simulink model "EN_EVPowerFlow_AveModel"  (R2021a)
settings: Solver=ode23t  StartTime=0.0  StopTime=20  MaxStep=1e-3  RelTol=1e-3  AbsTol=1e-3
libraries: nesl_utility x15, fl_lib x13, ee_lib x9, eeGeneralControl x4, pid_lib x1
settings Model: SimulationMode=accelerator  PacingRate=1000  Creator=ykamatan  LastModifiedBy=ykamatan
settings SolverCC: AutoScaleAbsTol=off  SolverJacobianMethodControl=SparsePerturbation  DaesscMode=Fast
settings DebuggingCC: SymbolicDimsDataTypeCodeGenerationDiagnostic=none  SFMachineParentedDataDiag=warning
settings SFSimCC: CustomCodeUndefinedFunction=UseInterfaceOnly
settings SimscapeCC: SimscapeLogType=all  SimscapeLogSimulationStatistics=on  SimscapeLogDataHistory=10000

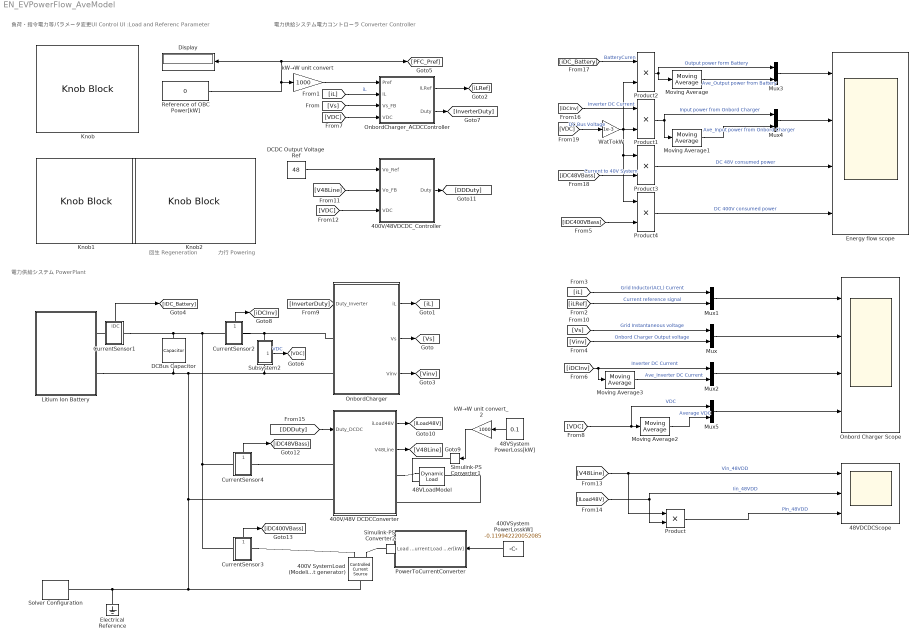
== system EN_EVPowerFlow_AveModel ==
  note: 回生
      | Regeneration
  note: 力行
      | Powering
  note: 負荷・指令電力等パラメータ変更UI
      | Control UI :Load and Referenc Parameter
  note: 電力供給システム PowerPlant
  note: 電力供給システム電力コントローラ
      | Converter Controller
  400V SystemLoad (Modeling as current generator) : fl_lib/Electrical/Electrical Sources/Controlled Current Source
  400V/48V DCDCConverter : Subsystem
  400V/48VDCDC_Controller : Subsystem
  400VSystem PowerLosskW] : Constant  Value=-0.119942220052085
  48VDCDCScope : Scope  NumInputPorts=3
  48VLoadModel : ee_lib/Passive/Dynamic Load  load_type=ee.enum.dc_ac.dc  enable_fault=ee.enum.faults.faultEnable.no  min_supply_voltage=38 V  pow_min=1e-3 W  G_reverse=1e-6 S  deltaV=1e-3 V  f0=60 Hz  Vrms_min=200 V  Pmin=1e-3 W  fault_action=ee.enum.faults.faultAction.none  t_fault=1 s  open_conductance=1e-4 S
      settings: SourceProductBaseCode=PS  InternalSimscapePortConfiguration="{\"Bottom\":[],\"Left\":[{\"id\":\"p\",\"label\":\"+\",\"type\":\"foundation.electrical.electrical\"}],\"Right\":[{\"id\":\"n\",\"label\":\"-\",\"type\":\"foundation.electrical.electrical\"}],\"Top\":[{\"id\":\"P\",\"label\":\"P\",\"type\":\"input\"}]}"
  48VSystem PowerLoss[kW] : Constant  Value=0.1
  CurrentSensor1 : Subsystem
      settings: PortSchema="{\"entries\":[{\"content\":{\"sides\":[{\"content\":{\"connectorIds\":[\"LConn1\"]},\"type\":\"ConnectorPlacement.EquallySpacedRectSide\",\"uuid\":\"7286f59e-cee0-499d-832c-cf6f33a1b017\"},{\"content\":{\"connectorIds\":[\"RConn1\"],\"side\":\"RIGHT\"},\"type\":\"ConnectorPlacement.EquallySpacedRectSide\",\"uuid\":\"6a983281-a6bc-4a57-a5ba-c4da9a8828f4\"},{\"content\":{\"connectorIds\":[\"Out1\"],\"side\":\"TOP\"},\"type\":\"ConnectorPlacement.EquallySpacedRectSide\",\"uuid\":\"6969f7e7-2dce-4d64-b6f6-e92ef9035b1a\"}]},\"type\":\"ConnectorPlacement.EquallySpacedConnector\",\"uuid\":\"05fc616a-5402-4b75-b59e-8cf259d71f3d\"}],\"packageUris\":[\"http://schema.mathworks.com/mf0/Connector/R2020b\"],\"version\":\"1.0\"}"
  CurrentSensor2 : Subsystem
      settings: PortSchema="{\"entries\":[{\"content\":{\"sides\":[{\"content\":{\"connectorIds\":[\"LConn1\"]},\"type\":\"ConnectorPlacement.EquallySpacedRectSide\",\"uuid\":\"7286f59e-cee0-499d-832c-cf6f33a1b017\"},{\"content\":{\"connectorIds\":[\"RConn1\"],\"side\":\"RIGHT\"},\"type\":\"ConnectorPlacement.EquallySpacedRectSide\",\"uuid\":\"6a983281-a6bc-4a57-a5ba-c4da9a8828f4\"},{\"content\":{\"connectorIds\":[\"Out1\"],\"side\":\"TOP\"},\"type\":\"ConnectorPlacement.EquallySpacedRectSide\",\"uuid\":\"6969f7e7-2dce-4d64-b6f6-e92ef9035b1a\"}]},\"type\":\"ConnectorPlacement.EquallySpacedConnector\",\"uuid\":\"05fc616a-5402-4b75-b59e-8cf259d71f3d\"}],\"packageUris\":[\"http://schema.mathworks.com/mf0/Connector/R2020b\"],\"version\":\"1.0\"}"
  CurrentSensor3 : Subsystem
      settings: PortSchema="{\"entries\":[{\"content\":{\"sides\":[{\"content\":{\"connectorIds\":[\"LConn1\"]},\"type\":\"ConnectorPlacement.EquallySpacedRectSide\",\"uuid\":\"7286f59e-cee0-499d-832c-cf6f33a1b017\"},{\"content\":{\"connectorIds\":[\"RConn1\"],\"side\":\"RIGHT\"},\"type\":\"ConnectorPlacement.EquallySpacedRectSide\",\"uuid\":\"6a983281-a6bc-4a57-a5ba-c4da9a8828f4\"},{\"content\":{\"connectorIds\":[\"Out1\"],\"side\":\"TOP\"},\"type\":\"ConnectorPlacement.EquallySpacedRectSide\",\"uuid\":\"6969f7e7-2dce-4d64-b6f6-e92ef9035b1a\"}]},\"type\":\"ConnectorPlacement.EquallySpacedConnector\",\"uuid\":\"05fc616a-5402-4b75-b59e-8cf259d71f3d\"}],\"packageUris\":[\"http://schema.mathworks.com/mf0/Connector/R2020b\"],\"version\":\"1.0\"}"
  CurrentSensor4 : Subsystem
      settings: PortSchema="{\"entries\":[{\"content\":{\"sides\":[{\"content\":{\"connectorIds\":[\"LConn1\"]},\"type\":\"ConnectorPlacement.EquallySpacedRectSide\",\"uuid\":\"7286f59e-cee0-499d-832c-cf6f33a1b017\"},{\"content\":{\"connectorIds\":[\"RConn1\"],\"side\":\"RIGHT\"},\"type\":\"ConnectorPlacement.EquallySpacedRectSide\",\"uuid\":\"6a983281-a6bc-4a57-a5ba-c4da9a8828f4\"},{\"content\":{\"connectorIds\":[\"Out1\"],\"side\":\"TOP\"},\"type\":\"ConnectorPlacement.EquallySpacedRectSide\",\"uuid\":\"6969f7e7-2dce-4d64-b6f6-e92ef9035b1a\"}]},\"type\":\"ConnectorPlacement.EquallySpacedConnector\",\"uuid\":\"05fc616a-5402-4b75-b59e-8cf259d71f3d\"}],\"packageUris\":[\"http://schema.mathworks.com/mf0/Connector/R2020b\"],\"version\":\"1.0\"}"
  DCBus Capacitor : ee_lib/Passive/Capacitor  cap_option=0  c=1000e-6 F  Cvec=[1e-05, 1e-06] F  Vvec=[0, 10] V  CV_table_symmetry=1  f_vec=[1, 10] kHz  DFext_vec=[.8, 1.2]  C_tol=5  enable_C_tol=0  tol_distribution=1  nSigma=4  r=1e-6 Ohm  g=0 1/Ohm  averaging_period=0 s  enable_operating_limits=0  operating_limit_action=2  max_working_voltage_range=[-25, 25] V  power_rating=1 W  enable_faults=0  fault_action=1  Cscale_faulted=100  R_faulted=1e-3 Ohm  G_faulted=0 1/Ohm  tau_fault=1e-3 s  enable_temporal_fault=0  t_fault=1 s  enable_behavioral_fault=0  max_permissible_voltage_range=[-100, 100] V  t_fail_on_voltage=1 s  i_specify=off  i_priority=None  i=0 A  i_nominal_specify=off  i_nominal_unit=A  i_nominal_value=1  v_specify=off  v_priority=None  v=400 V  v_nominal_specify=off  v_nominal_unit=V  v_nominal_value=1  vc_specify=on  vc_priority=High  vc=400 V  vc_nominal_specify=off  vc_nominal_unit=V  vc_nominal_value=1
  DCDC Output Voltage Ref : Constant  Value=48
  Display : Display
  Electrical Reference : fl_lib/Electrical/Electrical Elements/Electrical Reference
  Energy flow scope : Scope  NumInputPorts=4
  Knob : KnobBlock  ScaleMax=3
  Knob1 : KnobBlock  ScaleMin=0.1  ScaleMax=2
  Knob2 : KnobBlock  ScaleMin=-20  ScaleMax=20  TickInterval=2
  Litium Ion Battery : Subsystem
  Moving Average : eeGeneralControl/Moving Average  VariantControl=Variant1  LabelModeActiveChoice=Discrete  f=120  x0=0  Ts=1/120/10
      settings: SourceProductBaseCode=PS
  Moving Average1 : eeGeneralControl/Moving Average  VariantControl=Variant1  LabelModeActiveChoice=Discrete  f=120  x0=0  Ts=1/120/10
      settings: SourceProductBaseCode=PS
  Moving Average2 : eeGeneralControl/Moving Average  VariantControl=Variant1  LabelModeActiveChoice=Discrete  f=120  x0=400  Ts=1/120/10
      settings: SourceProductBaseCode=PS
  Moving Average3 : eeGeneralControl/Moving Average  VariantControl=Variant1  LabelModeActiveChoice=Discrete  f=120  x0=0  Ts=1/120/10
      settings: SourceProductBaseCode=PS
  Mux{,1..5} (6 alike) : Mux  Inputs=2
  Onbord Charger Scope : Scope  NumInputPorts=4
  OnbordCharger : Subsystem
  OnbordCharger_ACDCController : Subsystem
  PowerToCurrentConverter : Subsystem
  Product{,1..4} (5 alike) : Product
  Reference of OBC Power[kW] : Constant  Value=0
  Simulink-PS Converter1 : nesl_utility/Simulink-PS Converter  PhysicalDomain=network_engine_domain  SubClassName=ps_input  LeftPortType=input  RightPortType=output  PseudoPeriodic=off  Frequencies=[]  NoiseDistribution=none  NoiseParameters=[]  Unit=1  AffineConversion=off  FilteringAndDerivatives=provide  SimscapeFilterOrder=1  InputFilterTimeConstant=0.001  UdotUserProvided=0
      settings: SourceProductBaseCode=PW,SS
  Simulink-PS Converter2 : nesl_utility/Simulink-PS Converter  PhysicalDomain=network_engine_domain  SubClassName=ps_input  LeftPortType=input  RightPortType=output  PseudoPeriodic=off  Frequencies=[]  NoiseDistribution=none  NoiseParameters=[]  Unit=1  AffineConversion=off  FilteringAndDerivatives=provide  SimscapeFilterOrder=1  InputFilterTimeConstant=0.001  UdotUserProvided=0
      settings: SourceProductBaseCode=PW,SS
  Solver Configuration : nesl_utility/Solver Configuration  PhysicalDomain=network_engine_domain  SubClassName=solver  LeftPortType=input  RightPortType=generic  Tones=[]  Harmonics=[]  SimulateNoise=off  Profile=off  UseLocalSampling=off  EnableSwitchedLinearOptims=on  FrequencyDomain=off  UseCCode=off  RelTol=0.001  AbsTol=1e-06  MinStep=1e-09  ToWorkspace=off  RevertToSquareIcSolve=off  NumHomotopyIterations=100  PhasorMode=off  PhasorModeNumHarmonics=1  DoDC=off  ResidualTolerance=1e-09  UseLocalSolver=off  LocalSolverChoice=NE_BACKWARD_EULER_ADVANCER  LocalSolverSampleTime=0.001  DoFixedCost=off  MaxNonlinIter=3  MaxModeIter=2  ComputeImpulses=off  ImpulseIterations=2  LinearAlgebra=auto  EquationFormulation=NE_TIME_EF  DelaysMemoryBudget=1024  AutomaticFiltering=on  FilteringTimeConstant=0.001  PartitionStorageMethod=AS_NEEDED  PartitionMemoryBudget=1024  PartitionMethod=ROBUST
      settings: SourceProductBaseCode=PW,SS
  Subsystem2 : Subsystem
      settings: PortSchema="{\"entries\":[{\"content\":{\"sides\":[{\"content\":{\"connectorIds\":[\"Out1\"]},\"type\":\"ConnectorPlacement.EquallySpacedRectSide\",\"uuid\":\"7286f59e-cee0-499d-832c-cf6f33a1b017\"},{\"content\":{\"connectorIds\":[],\"side\":\"RIGHT\"},\"type\":\"ConnectorPlacement.EquallySpacedRectSide\",\"uuid\":\"6a983281-a6bc-4a57-a5ba-c4da9a8828f4\"},{\"content\":{\"connectorIds\":[\"LConn1\"],\"side\":\"TOP\"},\"type\":\"ConnectorPlacement.EquallySpacedRectSide\",\"uuid\":\"6969f7e7-2dce-4d64-b6f6-e92ef9035b1a\"},{\"content\":{\"connectorIds\":[\"RConn1\"],\"side\":\"BOTTOM\"},\"type\":\"ConnectorPlacement.EquallySpacedRectSide\",\"uuid\":\"8f7d22cd-967a-487e-912d-7270502758f1\"}]},\"type\":\"ConnectorPlacement.EquallySpacedConnector\",\"uuid\":\"05fc616a-5402-4b75-b59e-8cf259d71f3d\"}],\"packageUris\":[\"http://schema.mathworks.com/mf0/Connector/R2020b\"],\"version\":\"1.0\"}"
  WatTokW : Gain  Gain=1e-3
  kW→W unit convert : Gain  Gain=1000
  kW→W unit convert_2 : Gain  Gain=1000
  wires:
  Mux/1 -> Onbord Charger Scope/2
  Subsystem2/1(Vdc) -> [VDC]  "VDC"
  [iLRef] -> Mux1/2  "Current reference signal"
  Mux1/1 -> Onbord Charger Scope/1
  [iL] -> Mux1/1  "Grid Inductor(ACL) Current"
  [Vinv] -> Mux/2  "Onbord Charger Output voltage"
  Reference of OBC Power[kW]/1 -> kW→W unit convert/1, [PFC_Pref], Display/1
  [iDCInv] -> Moving Average3/1, Mux2/1  "Inverter DC Current"
  Mux2/1 -> Onbord Charger Scope/3
  Moving Average3/1 -> Mux2/2  "Ave_Inverter DC Current"
  [VDC] -> Mux5/1, Moving Average2/1  "VDC"
  [Vs] -> Mux/1  "Grid Instantaneous voltage"
  [iL] -> OnbordCharger_ACDCController/2(iL)  "iL"
  [Vs] -> OnbordCharger_ACDCController/3(Vs_FB)
  [VDC] -> OnbordCharger_ACDCController/4(VDC)
  OnbordCharger_ACDCController/1(iLRef) -> [iLRef]
  OnbordCharger_ACDCController/2(Duty) -> [InverterDuty]
  CurrentSensor2/1(iDCInv) -> [iDCInv]
  [V48Line] -> Product/1, 48VDCDCScope/1  "Vin_48VDD"
  [ILoad48V] -> Product/2, 48VDCDCScope/2  "Iin_48VDD"
  Product/1 -> 48VDCDCScope/3  "Pin_48VDD"
  Product1/1 -> Mux4/1, Moving Average1/1  "Input power from Onbord Charger"
  [iDC_Battery] -> Product2/1  "BatteryCuren"
  CurrentSensor4/1(iDC48VBass) -> [iDC48VBass]
  [iDC48VBass] -> Product3/2  "Current to 40V System"
  [iDCInv] -> Product1/1  "Inverter DC Current"
  [VDC] -> WatTokW/1  "DC Bus Voltage"
  Product2/1 -> Mux3/1, Moving Average/1  "Output power form Battery"
  Product3/1 -> Energy flow scope/3  "DC 48V consumed power"
  Mux3/1 -> Energy flow scope/1
  Moving Average/1 -> Mux3/2  "Ave_Output power from Battery"
  Mux4/1 -> Energy flow scope/2
  Moving Average1/1 -> Mux4/2  "Ave_Input power from Onbord Charger"
  Moving Average2/1 -> Mux5/2  "Average VDC"
  Mux5/1 -> Onbord Charger Scope/4
  [InverterDuty] -> OnbordCharger/1(Duty_Inverter)
  OnbordCharger/1(iL) -> [iL]
  OnbordCharger/2(Vs) -> [Vs]
  OnbordCharger/3(Vinv) -> [Vinv]
  [DDDuty] -> 400V/48V DCDCConverter/1(Duty_DCDC)
  400V/48V DCDCConverter/1(iLoad48V) -> [ILoad48V]
  400V/48V DCDCConverter/2(V48Line) -> [V48Line]
  CurrentSensor1/1(iDC) -> [iDC_Battery]
  DCDC Output Voltage Ref/1 -> 400V/48VDCDC_Controller/1(Vo_Ref)
  [V48Line] -> 400V/48VDCDC_Controller/2(Vo_FB)
  400V/48VDCDC_Controller/1(Duty) -> [DDDuty]
  [VDC] -> 400V/48VDCDC_Controller/3(VDC)
  CurrentSensor3/1(iDC400VBass) -> [iDC400VBass]
  [iDC400VBass] -> Product4/2
  Product4/1 -> Energy flow scope/4  "DC 400V consumed power"
  kW→W unit convert_2/1 -> Simulink-PS Converter1/1
  400VSystem PowerLosskW]/1 -> PowerToCurrentConverter/1(Load loss power[kW])
  PowerToCurrentConverter/1(Load Current) -> Simulink-PS Converter2/1
  kW→W unit convert/1 -> OnbordCharger_ACDCController/1(Pref)
  48VSystem PowerLoss[kW]/1 -> kW→W unit convert_2/1
  WatTokW/1 -> Product2/2, Product1/2, Product3/1, Product4/1
  connections:
  Subsystem2/LConn1 -- OnbordCharger/LConn1 -- CurrentSensor2/RConn1
  CurrentSensor2/LConn1 -- CurrentSensor3/LConn1 -- CurrentSensor4/LConn1 -- CurrentSensor1/RConn1 -- DCBus Capacitor/LConn1
  Simulink-PS Converter1/RConn1 -- 48VLoadModel/LConn2
  Litium Ion Battery/RConn2 -- 400V SystemLoad (Modeling as current generator)/LConn1 -- Electrical Reference/LConn1 -- Solver Configuration/RConn1 -- 400V/48V DCDCConverter/LConn2 -- OnbordCharger/LConn2 -- Subsystem2/RConn1 -- DCBus Capacitor/RConn1
  400V/48V DCDCConverter/RConn1 -- 48VLoadModel/LConn1
  CurrentSensor4/RConn1 -- 400V/48V DCDCConverter/LConn1
  48VLoadModel/RConn1 -- 400V/48V DCDCConverter/RConn2
  CurrentSensor1/LConn1 -- Litium Ion Battery/RConn1
  Simulink-PS Converter2/RConn1 -- 400V SystemLoad (Modeling as current generator)/RConn1
  CurrentSensor3/RConn1 -- 400V SystemLoad (Modeling as current generator)/RConn2

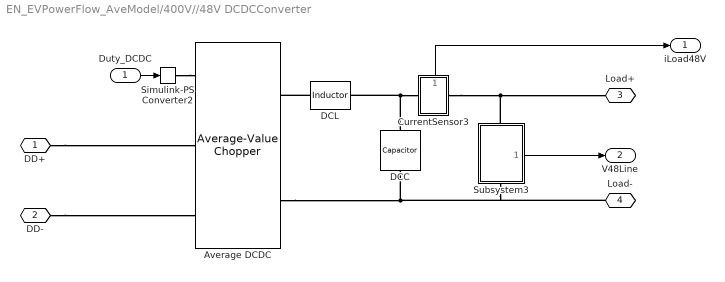
== system EN_EVPowerFlow_AveModel/400V//48V DCDCConverter ==
  Duty_DCDC : Inport
  Average DCDC : ee_lib/Semiconductors & Converters/Converters/Average-Value Chopper  chopper_type=5  efficiency_option=1  efficiency_fixed=100  i_vec=[0, 2, 5] A  efficiency_vec=[90, 95, 98]
      settings: SourceProductBaseCode=PS  InternalSimscapePortConfiguration="{\"Bottom\":[],\"Left\":[{\"id\":\"DutyCycle\",\"label\":\"DutyCycle\",\"type\":\"input\"},{\"id\":\"p1\",\"label\":\"1+\",\"type\":\"foundation.electrical.electrical\"},{\"id\":\"n1\",\"label\":\"1-\",\"type\":\"foundation.electrical.electrical\"}],\"Right\":[{\"id\":\"p2\",\"label\":\"2+\",\"type\":\"foundation.electrical.electrical\"},{\"id\":\"n2\",\"label\":\"2-\",\"type\":\"foundation.electrical.electrical\"}],\"Top\":[]}"
  CurrentSensor3 : Subsystem
      settings: PortSchema="{\"entries\":[{\"content\":{\"sides\":[{\"content\":{\"connectorIds\":[\"LConn1\"]},\"type\":\"ConnectorPlacement.EquallySpacedRectSide\",\"uuid\":\"7286f59e-cee0-499d-832c-cf6f33a1b017\"},{\"content\":{\"connectorIds\":[\"RConn1\"],\"side\":\"RIGHT\"},\"type\":\"ConnectorPlacement.EquallySpacedRectSide\",\"uuid\":\"6a983281-a6bc-4a57-a5ba-c4da9a8828f4\"},{\"content\":{\"connectorIds\":[\"Out1\"],\"side\":\"TOP\"},\"type\":\"ConnectorPlacement.EquallySpacedRectSide\",\"uuid\":\"6969f7e7-2dce-4d64-b6f6-e92ef9035b1a\"}]},\"type\":\"ConnectorPlacement.EquallySpacedConnector\",\"uuid\":\"05fc616a-5402-4b75-b59e-8cf259d71f3d\"}],\"packageUris\":[\"http://schema.mathworks.com/mf0/Connector/R2020b\"],\"version\":\"1.0\"}"
  DCC : ee_lib/Passive/Capacitor  cap_option=0  c=100e-6 F  Cvec=[1e-05, 1e-06] F  Vvec=[0, 10] V  CV_table_symmetry=1  f_vec=[1, 10] kHz  DFext_vec=[.8, 1.2]  C_tol=5  enable_C_tol=0  tol_distribution=1  nSigma=4  r=100e-3 Ohm  g=0 1/Ohm  averaging_period=0 s  enable_operating_limits=0  operating_limit_action=2  max_working_voltage_range=[-25, 25] V  power_rating=1 W  enable_faults=0  fault_action=1  Cscale_faulted=100  R_faulted=1e-3 Ohm  G_faulted=0 1/Ohm  tau_fault=1e-3 s  enable_temporal_fault=0  t_fault=1 s  enable_behavioral_fault=0  max_permissible_voltage_range=[-100, 100] V  t_fail_on_voltage=1 s  i_specify=off  i_priority=None  i=0 A  i_nominal_specify=off  i_nominal_unit=A  i_nominal_value=1  v_specify=off  v_priority=None  v=400 V  v_nominal_specify=off  v_nominal_unit=V  v_nominal_value=1  vc_specify=on  vc_priority=High  vc=48 V  vc_nominal_specify=off  vc_nominal_unit=V  vc_nominal_value=1
  DCL : ee_lib/Passive/Inductor  l=10e-6 H  L_tol=20  enable_L_tol=0  tol_distribution=1  nSigma=4  r=0.1 Ohm  g=1e-9 1/Ohm  enable_operating_limits=0  operating_limit_action=2  max_working_current=1 A  power_rating=1 W  enable_faults=0  fault_action=1  lambdaPercent=50  k_faulted=0.9999  turnsShort=0  openCct=0  groundShort=0  groundShortG=0 1/Ohm  tau_fault=1e-3 s  enable_temporal_fault=0  t_fault=1 s  enable_behavioral_fault=0  max_permissible_voltage=100 V  n_fail_on_voltage=1  max_permissible_current=1 A  t_fail_on_current=1 s  i_L_specify=off  i_L_priority=High  i_L=0 A  i_L_nominal_specify=off  i_L_nominal_unit=A  i_L_nominal_value=1
  Simulink-PS Converter2 : nesl_utility/Simulink-PS Converter  PhysicalDomain=network_engine_domain  SubClassName=ps_input  LeftPortType=input  RightPortType=output  PseudoPeriodic=off  Frequencies=[]  NoiseDistribution=none  NoiseParameters=[]  Unit=1  AffineConversion=off  FilteringAndDerivatives=provide  SimscapeFilterOrder=1  InputFilterTimeConstant=0.001  UdotUserProvided=0
      settings: SourceProductBaseCode=PW,SS
  Subsystem3 : Subsystem
      settings: PortSchema="{\"entries\":[{\"content\":{\"sides\":[{\"content\":{\"connectorIds\":[]},\"type\":\"ConnectorPlacement.EquallySpacedRectSide\",\"uuid\":\"7286f59e-cee0-499d-832c-cf6f33a1b017\"},{\"content\":{\"connectorIds\":[\"Out1\"],\"side\":\"RIGHT\"},\"type\":\"ConnectorPlacement.EquallySpacedRectSide\",\"uuid\":\"6a983281-a6bc-4a57-a5ba-c4da9a8828f4\"},{\"content\":{\"connectorIds\":[\"LConn1\"],\"side\":\"TOP\"},\"type\":\"ConnectorPlacement.EquallySpacedRectSide\",\"uuid\":\"6969f7e7-2dce-4d64-b6f6-e92ef9035b1a\"},{\"content\":{\"connectorIds\":[\"RConn1\"],\"side\":\"BOTTOM\"},\"type\":\"ConnectorPlacement.EquallySpacedRectSide\",\"uuid\":\"8f7d22cd-967a-487e-912d-7270502758f1\"}]},\"type\":\"ConnectorPlacement.EquallySpacedConnector\",\"uuid\":\"05fc616a-5402-4b75-b59e-8cf259d71f3d\"}],\"packageUris\":[\"http://schema.mathworks.com/mf0/Connector/R2020b\"],\"version\":\"1.0\"}"
  DD+ : PMIOPort  Side=Left
  DD- : PMIOPort  Port=2  Side=Left
  Load+ : PMIOPort  Port=3  Side=Right
  Load- : PMIOPort  Port=4  Side=Right
  iLoad48V : Outport
  V48Line : Outport  Port=2
  wires:
  Duty_DCDC/1 -> Simulink-PS Converter2/1
  Subsystem3/1(V48Line) -> V48Line/1
  CurrentSensor3/1(iLoad48V) -> iLoad48V/1
  connections:
  Simulink-PS Converter2/RConn1 -- Average DCDC/LConn1
  Average DCDC/RConn2 -- Subsystem3/RConn1 -- Load-/RConn1 -- DCC/RConn1
  DD-/RConn1 -- Average DCDC/LConn3
  DCC/LConn1 -- CurrentSensor3/LConn1 -- DCL/RConn1
  DCL/LConn1 -- Average DCDC/RConn1
  Subsystem3/LConn1 -- Load+/RConn1 -- CurrentSensor3/RConn1
  DD+/RConn1 -- Average DCDC/LConn2

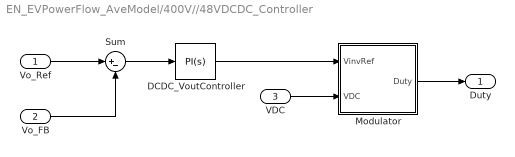
== system EN_EVPowerFlow_AveModel/400V//48VDCDC_Controller ==
  Vo_Ref : Inport
  Vo_FB : Inport  Port=2
  VDC : Inport  Port=3
  DCDC_VoutController : pid_lib/PID Controller  Controller=PI  Form=Parallel  TimeDomain=Continuous-time  UseExternalTs=off  SampleTime=-1  IntegratorMethod=Forward Euler  FilterMethod=Forward Euler  ControllerParametersSource=internal  P=0.05  I=70  D=0.00044655786441046  UseFilter=on  N=150907.276527032  TunerSelectOption=Transfer Function Based (PID Tuner App)  InitialConditionSource=internal  InitialConditionForIntegrator=0  InitialConditionForFilter=0  DifferentiatorICPrevScaledInput=0  ExternalReset=none  TrackingMode=off  Kt=1  LimitOutput=off  SatLimitsSource=internal  UpperSaturationLimit=inf  LowerSaturationLimit=-inf  LinearizeAsGain=on  AntiWindupMode=none  Kb=1  POutMin=[]  POutMax=[]  IOutMin=[]  IOutMax=[]  DOutMin=[]  DOutMax=[]  NOutMin=[]  NOutMax=[]  SumOutMin=[]  SumOutMax=[]  SaturationOutMin=[]  SaturationOutMax=[]  PParamMin=[]  PParamMax=[]  IParamMin=[]  IParamMax=[]  DParamMin=[]  DParamMax=[]  NParamMin=[]  NParamMax=[]  KbParamMin=[]  KbParamMax=[]  KtParamMin=[]  KtParamMax=[]  KbOutMin=[]  KbOutMax=[]  KtOutMin=[]  KtOutMax=[]  IntegratorOutMin=[]  IntegratorOutMax=[]  FilterOutMin=[]  FilterOutMax=[]  SumI1OutMin=[]  SumI1OutMax=[]  SumI2OutMin=[]  SumI2OutMax=[]  SumI3OutMin=[]  SumI3OutMax=[]  SumI4OutMin=[]  SumI4OutMax=[]  SumDOutMin=[]  SumDOutMax=[]  DifferentiatorOutMin=[]  DifferentiatorOutMax=[]  FilterDiffOutCoefMin=[]  FilterDiffOutCoefMax=[]  ReciprocalOutMin=[]  ReciprocalOutMax=[]  SumDenOutMin=[]  SumDenOutMax=[]  SumNumOutMin=[]  SumNumOutMax=[]  DivideOutMin=[]  DivideOutMax=[]  UdiffTsProdOutMin=[]  UdiffTsProdOutMax=[]  NTsProdOutMin=[]  NTsProdOutMax=[]  UintegralTsProdOutMin=[]  UintegralTsProdOutMax=[]  UngainTsProdOutMin=[]  UngainTsProdOutMax=[]  IntegratorContinuousStateAttributes=''  IntegratorStateMustResolveToSignalObject=off  IntegratorRTWStateStorageClass=Auto  FilterContinuousStateAttributes=''  FilterStateMustResolveToSignalObject=off  FilterRTWStateStorageClass=Auto  ParallelPVariant=InternalParameters  IdealPVariant=Disabled  IVariant=InternalParameters  DVariant=Disabled  IntegratorVariant=Continuous  SatVariant=Disabled  AWVariant=Passthrough  PCopyVariant=Disabled  TRVariant=Disabled  FdbkBlocksVariant=Forward  IdealPFdbkVariant=Disabled  SatFdbkVariant=Disabled  DerivativeFilterVariant=Disabled  NVariant=Disabled  NCopyVariant=Disabled_SignalSpec  FilterICVariant=Disabled  IntegratorICVariant=InternalICs  ExternalResetVariant=Disabled  TRSumVariant=Passthrough  SumFdbkVariant=Disabled  SumVariant=Sum_PI  TsampFilterVariant=InternalTs  TsampNgainVariant=Passthrough  TsampIntegralVariant=Passthrough  ExternalSaturationOutDataTypeStr=Inherit: Same as second input
  Modulator : Subsystem
  Sum : Sum  Inputs=|+-
  Duty : Outport
  wires:
  Sum/1 -> DCDC_VoutController/1
  Vo_FB/1 -> Sum/2
  DCDC_VoutController/1 -> Modulator/1(VinvRef)
  VDC/1 -> Modulator/2(VDC)
  Modulator/1(Duty) -> Duty/1
  Vo_Ref/1 -> Sum/1

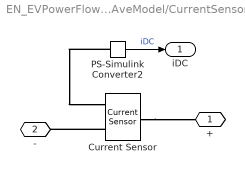
== system EN_EVPowerFlow_AveModel/CurrentSensor1 ==
  Current Sensor : fl_lib/Electrical/Electrical Sensors/Current Sensor
  PS-Simulink Converter2 : nesl_utility/PS-Simulink Converter  PhysicalDomain=network_engine_domain  SubClassName=ps_output  LeftPortType=input  RightPortType=output  PseudoPeriodic=off  Frequencies=[]  Unit=inherit  AffineConversion=off
      settings: SourceProductBaseCode=PW,SS
  + : PMIOPort  Side=Left
  - : PMIOPort  Port=2  Side=Right
  iDC : Outport
  wires:
  PS-Simulink Converter2/1 -> iDC/1  "iDC"
  connections:
  Current Sensor/LConn1 -- +/RConn1
  PS-Simulink Converter2/LConn1 -- Current Sensor/RConn1
  Current Sensor/RConn2 -- -/RConn1

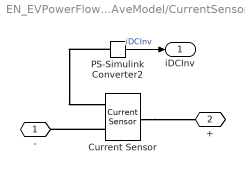
== system EN_EVPowerFlow_AveModel/CurrentSensor2 ==
  Current Sensor : fl_lib/Electrical/Electrical Sensors/Current Sensor
  PS-Simulink Converter2 : nesl_utility/PS-Simulink Converter  PhysicalDomain=network_engine_domain  SubClassName=ps_output  LeftPortType=input  RightPortType=output  PseudoPeriodic=off  Frequencies=[]  Unit=inherit  AffineConversion=off
      settings: SourceProductBaseCode=PW,SS
  - : PMIOPort  Side=Left
  + : PMIOPort  Port=2  Side=Right
  iDCInv : Outport
  wires:
  PS-Simulink Converter2/1 -> iDCInv/1  "iDCInv"
  connections:
  Current Sensor/LConn1 -- +/RConn1
  PS-Simulink Converter2/LConn1 -- Current Sensor/RConn1
  Current Sensor/RConn2 -- -/RConn1

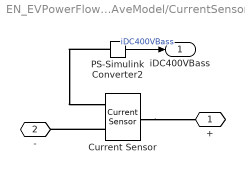
== system EN_EVPowerFlow_AveModel/CurrentSensor3 ==
  Current Sensor : fl_lib/Electrical/Electrical Sensors/Current Sensor
  PS-Simulink Converter2 : nesl_utility/PS-Simulink Converter  PhysicalDomain=network_engine_domain  SubClassName=ps_output  LeftPortType=input  RightPortType=output  PseudoPeriodic=off  Frequencies=[]  Unit=inherit  AffineConversion=off
      settings: SourceProductBaseCode=PW,SS
  + : PMIOPort  Side=Left
  - : PMIOPort  Port=2  Side=Right
  iDC400VBass : Outport
  wires:
  PS-Simulink Converter2/1 -> iDC400VBass/1  "iDC400VBass"
  connections:
  Current Sensor/LConn1 -- +/RConn1
  PS-Simulink Converter2/LConn1 -- Current Sensor/RConn1
  Current Sensor/RConn2 -- -/RConn1

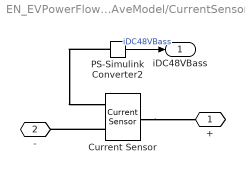
== system EN_EVPowerFlow_AveModel/CurrentSensor4 ==
  Current Sensor : fl_lib/Electrical/Electrical Sensors/Current Sensor
  PS-Simulink Converter2 : nesl_utility/PS-Simulink Converter  PhysicalDomain=network_engine_domain  SubClassName=ps_output  LeftPortType=input  RightPortType=output  PseudoPeriodic=off  Frequencies=[]  Unit=inherit  AffineConversion=off
      settings: SourceProductBaseCode=PW,SS
  + : PMIOPort  Side=Left
  - : PMIOPort  Port=2  Side=Right
  iDC48VBass : Outport
  wires:
  PS-Simulink Converter2/1 -> iDC48VBass/1  "iDC48VBass"
  connections:
  Current Sensor/LConn1 -- +/RConn1
  PS-Simulink Converter2/LConn1 -- Current Sensor/RConn1
  Current Sensor/RConn2 -- -/RConn1

== system EN_EVPowerFlow_AveModel/Litium Ion Battery ==
  400V Nominal Battery : ee_lib/Sources/Battery  Vnom=400 V  prm_dir=1  R1_dis=2 Ohm  R1_ch=2 Ohm  R1=1 Ohm  prm_AH=2  AH=0.5 hr*A  V1=380 V  AH1=0.25 hr*A  prm_R2=1  R2=2000 Ohm  prm_dyn=2  Rp1=0.05 Ohm  tau1=30 s  Rp2=0.005 Ohm  tau2=30 s  Rp3=0.005 Ohm  tau3=30 s  Rp4=0.005 Ohm  tau4=30 s  Rp5=0.005 Ohm  tau5=30 s  prm_fade=1  N_fade=100  AH_fade=45 hr*A  R1_fade=2.02 Ohm  R1_ch_fade=2.02 Ohm  V1_fade=10.35 V  prm_age=1  prm_age_OCV=1  OCV_age=0.9  SOC_age=60  Tmeas_age=298.15 K  delta_time_age_vec=[0] d  temperature_age_vec=[273] K  OCV_scaling_age=2.2134e6  OCV_offset_age=1.632e6  temp_exp_age=0.515833569 V  t_exp_age=0.75  i_specify=off  i_priority=None  i=0 A  i_nominal_specify=off  i_nominal_unit=A  i_nominal_value=1  v_specify=off  v_priority=None  v=0 V  v_nominal_specify=off  v_nominal_unit=V  v_nominal_value=1  charge_specify=on  charge_priority=High  charge=0.25 hr*A  charge_nominal_specify=off  charge_nominal_unit=hr*A  charge_nominal_value=1  num_cycles_specify=off  num_cycles_priority=High  num_cycles=0  num_cycles_nominal_specify=off  num_cycles_nominal_unit=1  num_cycles_nominal_value=1  thermal_mass=30000 J/K  Tmeas=298.15 K  Vnom_T2=12 V  R1_T2=2.2 Ohm  R1_T2_dis=2.2 Ohm  R1_T2_ch=2.2 Ohm  V1_T2=11.4 V  R2_T2=2200 Ohm  Rp1_T2=0.005 Ohm  tau1_T2=30 s  Rp2_T2=0.005 Ohm  tau2_T2=30 s  Rp3_T2=0.005 Ohm  tau3_T2=30 s  Rp4_T2=0.005 Ohm  tau4_T2=30 s  Rp5_T2=0.005 Ohm  tau5_T2=30 s  Tmeas2=273.15 K  temperature_specify=off  temperature_priority=High  temperature=298.15 K  temperature_nominal_specify=off  temperature_nominal_unit=K  temperature_nominal_value=1
  Bat+ : PMIOPort  Side=Right
  Bat- : PMIOPort  Port=2  Side=Right
  connections:
  Bat+/RConn1 -- 400V Nominal Battery/LConn1
  400V Nominal Battery/RConn1 -- Bat-/RConn1

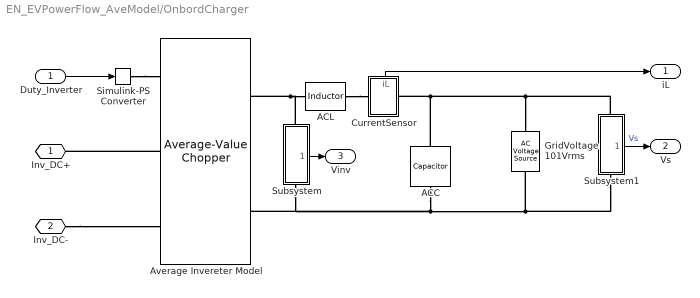
== system EN_EVPowerFlow_AveModel/OnbordCharger ==
  Duty_Inverter : Inport
  ACC : ee_lib/Passive/Capacitor  cap_option=0  c=10e-6 F  Cvec=[1e-05, 1e-06] F  Vvec=[0, 10] V  CV_table_symmetry=1  f_vec=[1, 10] kHz  DFext_vec=[.8, 1.2]  C_tol=5  enable_C_tol=0  tol_distribution=1  nSigma=4  r=100e-3 Ohm  g=0 1/Ohm  averaging_period=0 s  enable_operating_limits=0  operating_limit_action=2  max_working_voltage_range=[-25, 25] V  power_rating=1 W  enable_faults=0  fault_action=1  Cscale_faulted=100  R_faulted=1e-3 Ohm  G_faulted=0 1/Ohm  tau_fault=1e-3 s  enable_temporal_fault=0  t_fault=1 s  enable_behavioral_fault=0  max_permissible_voltage_range=[-100, 100] V  t_fail_on_voltage=1 s  i_specify=off  i_priority=None  i=0 A  i_nominal_specify=off  i_nominal_unit=A  i_nominal_value=1  v_specify=off  v_priority=None  v=400 V  v_nominal_specify=off  v_nominal_unit=V  v_nominal_value=1  vc_specify=off  vc_priority=High  vc=48 V  vc_nominal_specify=off  vc_nominal_unit=V  vc_nominal_value=1
  ACL : ee_lib/Passive/Inductor  l=1e-3 H  L_tol=20  enable_L_tol=0  tol_distribution=1  nSigma=4  r=0.1 Ohm  g=1e-9 1/Ohm  enable_operating_limits=0  operating_limit_action=2  max_working_current=1 A  power_rating=1 W  enable_faults=0  fault_action=1  lambdaPercent=50  k_faulted=0.9999  turnsShort=0  openCct=0  groundShort=0  groundShortG=0 1/Ohm  tau_fault=1e-3 s  enable_temporal_fault=0  t_fault=1 s  enable_behavioral_fault=0  max_permissible_voltage=100 V  n_fail_on_voltage=1  max_permissible_current=1 A  t_fail_on_current=1 s  i_L_specify=off  i_L_priority=High  i_L=0 A  i_L_nominal_specify=off  i_L_nominal_unit=A  i_L_nominal_value=1
  Average Invereter Model : ee_lib/Semiconductors & Converters/Converters/Average-Value Chopper  chopper_type=5  efficiency_option=1  efficiency_fixed=100  i_vec=[0, 2, 5] A  efficiency_vec=[90, 95, 98]
      settings: SourceProductBaseCode=PS  InternalSimscapePortConfiguration="{\"Bottom\":[],\"Left\":[{\"id\":\"DutyCycle\",\"label\":\"DutyCycle\",\"type\":\"input\"},{\"id\":\"p1\",\"label\":\"1+\",\"type\":\"foundation.electrical.electrical\"},{\"id\":\"n1\",\"label\":\"1-\",\"type\":\"foundation.electrical.electrical\"}],\"Right\":[{\"id\":\"p2\",\"label\":\"2+\",\"type\":\"foundation.electrical.electrical\"},{\"id\":\"n2\",\"label\":\"2-\",\"type\":\"foundation.electrical.electrical\"}],\"Top\":[]}"
  CurrentSensor : Subsystem
      settings: PortSchema="{\"entries\":[{\"content\":{\"sides\":[{\"content\":{\"connectorIds\":[\"LConn1\"]},\"type\":\"ConnectorPlacement.EquallySpacedRectSide\",\"uuid\":\"7286f59e-cee0-499d-832c-cf6f33a1b017\"},{\"content\":{\"connectorIds\":[\"RConn1\"],\"side\":\"RIGHT\"},\"type\":\"ConnectorPlacement.EquallySpacedRectSide\",\"uuid\":\"6a983281-a6bc-4a57-a5ba-c4da9a8828f4\"},{\"content\":{\"connectorIds\":[\"Out1\"],\"side\":\"TOP\"},\"type\":\"ConnectorPlacement.EquallySpacedRectSide\",\"uuid\":\"6969f7e7-2dce-4d64-b6f6-e92ef9035b1a\"}]},\"type\":\"ConnectorPlacement.EquallySpacedConnector\",\"uuid\":\"05fc616a-5402-4b75-b59e-8cf259d71f3d\"}],\"packageUris\":[\"http://schema.mathworks.com/mf0/Connector/R2020b\"],\"version\":\"1.0\"}"
  GridVoltage 101Vrms : fl_lib/Electrical/Electrical Sources/AC Voltage Source  amp=101*1.414 V  shift=0 deg  frequency=60 Hz  omega=0 rad/s
  Simulink-PS Converter : nesl_utility/Simulink-PS Converter  PhysicalDomain=network_engine_domain  SubClassName=ps_input  LeftPortType=input  RightPortType=output  PseudoPeriodic=off  Frequencies=[]  NoiseDistribution=none  NoiseParameters=[]  Unit=1  AffineConversion=off  FilteringAndDerivatives=provide  SimscapeFilterOrder=1  InputFilterTimeConstant=0.001  UdotUserProvided=0
      settings: SourceProductBaseCode=PW,SS
  Subsystem : Subsystem
      settings: PortSchema="{\"entries\":[{\"content\":{\"sides\":[{\"content\":{\"connectorIds\":[]},\"type\":\"ConnectorPlacement.EquallySpacedRectSide\",\"uuid\":\"7286f59e-cee0-499d-832c-cf6f33a1b017\"},{\"content\":{\"connectorIds\":[\"Out1\"],\"side\":\"RIGHT\"},\"type\":\"ConnectorPlacement.EquallySpacedRectSide\",\"uuid\":\"6a983281-a6bc-4a57-a5ba-c4da9a8828f4\"},{\"content\":{\"connectorIds\":[\"LConn1\"],\"side\":\"TOP\"},\"type\":\"ConnectorPlacement.EquallySpacedRectSide\",\"uuid\":\"6969f7e7-2dce-4d64-b6f6-e92ef9035b1a\"},{\"content\":{\"connectorIds\":[\"RConn1\"],\"side\":\"BOTTOM\"},\"type\":\"ConnectorPlacement.EquallySpacedRectSide\",\"uuid\":\"8f7d22cd-967a-487e-912d-7270502758f1\"}]},\"type\":\"ConnectorPlacement.EquallySpacedConnector\",\"uuid\":\"05fc616a-5402-4b75-b59e-8cf259d71f3d\"}],\"packageUris\":[\"http://schema.mathworks.com/mf0/Connector/R2020b\"],\"version\":\"1.0\"}"
  Subsystem1 : Subsystem
      settings: PortSchema="{\"entries\":[{\"content\":{\"sides\":[{\"content\":{\"connectorIds\":[]},\"type\":\"ConnectorPlacement.EquallySpacedRectSide\",\"uuid\":\"7286f59e-cee0-499d-832c-cf6f33a1b017\"},{\"content\":{\"connectorIds\":[\"Out1\"],\"side\":\"RIGHT\"},\"type\":\"ConnectorPlacement.EquallySpacedRectSide\",\"uuid\":\"6a983281-a6bc-4a57-a5ba-c4da9a8828f4\"},{\"content\":{\"connectorIds\":[\"LConn1\"],\"side\":\"TOP\"},\"type\":\"ConnectorPlacement.EquallySpacedRectSide\",\"uuid\":\"6969f7e7-2dce-4d64-b6f6-e92ef9035b1a\"},{\"content\":{\"connectorIds\":[\"RConn1\"],\"side\":\"BOTTOM\"},\"type\":\"ConnectorPlacement.EquallySpacedRectSide\",\"uuid\":\"8f7d22cd-967a-487e-912d-7270502758f1\"}]},\"type\":\"ConnectorPlacement.EquallySpacedConnector\",\"uuid\":\"05fc616a-5402-4b75-b59e-8cf259d71f3d\"}],\"packageUris\":[\"http://schema.mathworks.com/mf0/Connector/R2020b\"],\"version\":\"1.0\"}"
  Inv_DC+ : PMIOPort  Side=Left
  Inv_DC- : PMIOPort  Port=2  Side=Left
  iL : Outport
  Vs : Outport  Port=2
  Vinv : Outport  Port=3
  wires:
  Duty_Inverter/1 -> Simulink-PS Converter/1
  CurrentSensor/1(iL) -> iL/1
  Subsystem/1(Vinv) -> Vinv/1
  Subsystem1/1(Vs) -> Vs/1  "Vs"
  connections:
  ACL/RConn1 -- CurrentSensor/LConn1
  Subsystem1/RConn1 -- Average Invereter Model/RConn2 -- Subsystem/RConn1 -- ACC/RConn1 -- GridVoltage 101Vrms/RConn1
  Subsystem/LConn1 -- Average Invereter Model/RConn1 -- ACL/LConn1
  Subsystem1/LConn1 -- ACC/LConn1 -- CurrentSensor/RConn1 -- GridVoltage 101Vrms/LConn1
  Simulink-PS Converter/RConn1 -- Average Invereter Model/LConn1
  Inv_DC-/RConn1 -- Average Invereter Model/LConn3
  Average Invereter Model/LConn2 -- Inv_DC+/RConn1

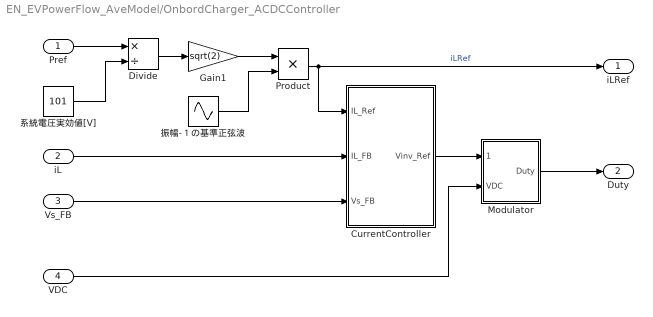
== system EN_EVPowerFlow_AveModel/OnbordCharger_ACDCController ==
  Pref : Inport
  iL : Inport  Port=2
  Vs_FB : Inport  Port=3
  VDC : Inport  Port=4
  CurrentController : Subsystem
  Divide : Product  Inputs=*/
  Gain1 : Gain  Gain=sqrt(2)
  Modulator : Subsystem
  Product : Product
  振幅-１の基準正弦波 : Sin  Amplitude=-1  Frequency=2*pi*60  SampleTime=0
  系統電圧実効値[V] : Constant  Value=101
  iLRef : Outport
  Duty : Outport  Port=2
  wires:
  iL/1 -> CurrentController/2(IL_FB)
  Pref/1 -> Divide/1
  Product/1 -> CurrentController/1(IL_Ref), iLRef/1  "iLRef"
  振幅-１の基準正弦波/1 -> Product/2
  Gain1/1 -> Product/1
  Vs_FB/1 -> CurrentController/3(Vs_FB)
  CurrentController/1(Vinv_Ref) -> Modulator/1(VinvRef)
  VDC/1 -> Modulator/2(VDC)
  Modulator/1(Duty) -> Duty/1
  Divide/1 -> Gain1/1
  系統電圧実効値[V]/1 -> Divide/2

== system EN_EVPowerFlow_AveModel/PowerToCurrentConverter ==
  Load loss power[kW] : Inport
  DCBus Typ Voltage : Constant  Value=400
  Divide : Product  Inputs=*/
  kW→W unit convert : Gain  Gain=1000
  Load Current : Outport
  wires:
  Load loss power[kW]/1 -> kW→W unit convert/1
  kW→W unit convert/1 -> Divide/1
  DCBus Typ Voltage/1 -> Divide/2
  Divide/1 -> Load Current/1

== system EN_EVPowerFlow_AveModel/Subsystem2 ==
  PS-Simulink Converter1 : nesl_utility/PS-Simulink Converter  PhysicalDomain=network_engine_domain  SubClassName=ps_output  LeftPortType=input  RightPortType=output  PseudoPeriodic=off  Frequencies=[]  Unit=inherit  AffineConversion=off
      settings: SourceProductBaseCode=PW,SS
  Voltage Sensor1 : fl_lib/Electrical/Electrical Sensors/Voltage Sensor
  + : PMIOPort  Side=Left
  - : PMIOPort  Port=2  Side=Right
  Vdc : Outport
  wires:
  PS-Simulink Converter1/1 -> Vdc/1  "Vdc"
  connections:
  Voltage Sensor1/RConn1 -- PS-Simulink Converter1/LConn1
  Voltage Sensor1/LConn1 -- +/RConn1
  Voltage Sensor1/RConn2 -- -/RConn1

== system EN_EVPowerFlow_AveModel/400V//48V DCDCConverter/CurrentSensor3 ==
  Current Sensor : fl_lib/Electrical/Electrical Sensors/Current Sensor
  PS-Simulink Converter2 : nesl_utility/PS-Simulink Converter  PhysicalDomain=network_engine_domain  SubClassName=ps_output  LeftPortType=input  RightPortType=output  PseudoPeriodic=off  Frequencies=[]  Unit=inherit  AffineConversion=off
      settings: SourceProductBaseCode=PW,SS
  + : PMIOPort  Side=Left
  - : PMIOPort  Port=2  Side=Right
  iLoad48V : Outport
  wires:
  PS-Simulink Converter2/1 -> iLoad48V/1  "iLoad48V"
  connections:
  Current Sensor/LConn1 -- +/RConn1
  PS-Simulink Converter2/LConn1 -- Current Sensor/RConn1
  Current Sensor/RConn2 -- -/RConn1

== system EN_EVPowerFlow_AveModel/400V//48V DCDCConverter/Subsystem3 ==
  PS-Simulink Converter1 : nesl_utility/PS-Simulink Converter  PhysicalDomain=network_engine_domain  SubClassName=ps_output  LeftPortType=input  RightPortType=output  PseudoPeriodic=off  Frequencies=[]  Unit=inherit  AffineConversion=off
      settings: SourceProductBaseCode=PW,SS
  Voltage Sensor1 : fl_lib/Electrical/Electrical Sensors/Voltage Sensor
  + : PMIOPort  Side=Left
  - : PMIOPort  Port=2  Side=Right
  V48Line : Outport
  wires:
  PS-Simulink Converter1/1 -> V48Line/1  "V48Line"
  connections:
  Voltage Sensor1/RConn1 -- PS-Simulink Converter1/LConn1
  Voltage Sensor1/LConn1 -- +/RConn1
  Voltage Sensor1/RConn2 -- -/RConn1

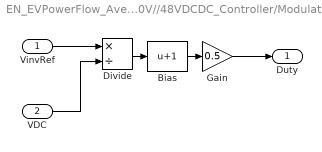
== system EN_EVPowerFlow_AveModel/400V//48VDCDC_Controller/Modulator ==
  VinvRef : Inport
  VDC : Inport  Port=2
  Bias : Bias  Bias=1
  Divide : Product  Inputs=*/
  Gain : Gain  Gain=0.5
  Duty : Outport
  wires:
  VDC/1 -> Divide/2
  Gain/1 -> Duty/1
  Divide/1 -> Bias/1
  Bias/1 -> Gain/1
  VinvRef/1 -> Divide/1

== system EN_EVPowerFlow_AveModel/OnbordCharger/CurrentSensor ==
  Current Sensor : fl_lib/Electrical/Electrical Sensors/Current Sensor
  PS-Simulink Converter2 : nesl_utility/PS-Simulink Converter  PhysicalDomain=network_engine_domain  SubClassName=ps_output  LeftPortType=input  RightPortType=output  PseudoPeriodic=off  Frequencies=[]  Unit=inherit  AffineConversion=off
      settings: SourceProductBaseCode=PW,SS
  + : PMIOPort  Side=Left
  - : PMIOPort  Port=2  Side=Right
  iL : Outport
  wires:
  PS-Simulink Converter2/1 -> iL/1  "iL"
  connections:
  Current Sensor/LConn1 -- +/RConn1
  PS-Simulink Converter2/LConn1 -- Current Sensor/RConn1
  Current Sensor/RConn2 -- -/RConn1

== system EN_EVPowerFlow_AveModel/OnbordCharger/Subsystem ==
  PS-Simulink Converter1 : nesl_utility/PS-Simulink Converter  PhysicalDomain=network_engine_domain  SubClassName=ps_output  LeftPortType=input  RightPortType=output  PseudoPeriodic=off  Frequencies=[]  Unit=inherit  AffineConversion=off
      settings: SourceProductBaseCode=PW,SS
  Voltage Sensor1 : fl_lib/Electrical/Electrical Sensors/Voltage Sensor
  + : PMIOPort  Side=Left
  - : PMIOPort  Port=2  Side=Right
  Vinv : Outport
  wires:
  PS-Simulink Converter1/1 -> Vinv/1  "Vinv"
  connections:
  Voltage Sensor1/RConn1 -- PS-Simulink Converter1/LConn1
  Voltage Sensor1/LConn1 -- +/RConn1
  Voltage Sensor1/RConn2 -- -/RConn1

== system EN_EVPowerFlow_AveModel/OnbordCharger/Subsystem1 ==
  PS-Simulink Converter1 : nesl_utility/PS-Simulink Converter  PhysicalDomain=network_engine_domain  SubClassName=ps_output  LeftPortType=input  RightPortType=output  PseudoPeriodic=off  Frequencies=[]  Unit=inherit  AffineConversion=off
      settings: SourceProductBaseCode=PW,SS
  Voltage Sensor1 : fl_lib/Electrical/Electrical Sensors/Voltage Sensor
  + : PMIOPort  Side=Left
  - : PMIOPort  Port=2  Side=Right
  Vs : Outport
  wires:
  PS-Simulink Converter1/1 -> Vs/1  "Vs"
  connections:
  Voltage Sensor1/RConn1 -- PS-Simulink Converter1/LConn1
  Voltage Sensor1/LConn1 -- +/RConn1
  Voltage Sensor1/RConn2 -- -/RConn1

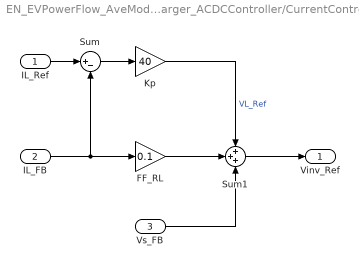
== system EN_EVPowerFlow_AveModel/OnbordCharger_ACDCController/CurrentController ==
  IL_Ref : Inport
  IL_FB : Inport  Port=2
  Vs_FB : Inport  Port=3
  FF_RL : Gain  Gain=0.1
  Kp : Gain  Gain=40
  Sum : Sum  Inputs=|+-
  Sum1 : Sum  Inputs=+++
  Vinv_Ref : Outport
  wires:
  IL_FB/1 -> FF_RL/1, Sum/2
  Kp/1 -> Sum1/1  "VL_Ref"
  Sum/1 -> Kp/1
  IL_Ref/1 -> Sum/1
  Vs_FB/1 -> Sum1/3
  Sum1/1 -> Vinv_Ref/1
  FF_RL/1 -> Sum1/2

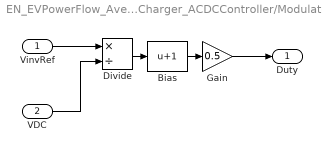
== system EN_EVPowerFlow_AveModel/OnbordCharger_ACDCController/Modulator ==
  VinvRef : Inport
  VDC : Inport  Port=2
  Bias : Bias  Bias=1
  Divide : Product  Inputs=*/
  Gain : Gain  Gain=0.5
  Duty : Outport
  wires:
  VDC/1 -> Divide/2
  Gain/1 -> Duty/1
  Divide/1 -> Bias/1
  Bias/1 -> Gain/1
  VinvRef/1 -> Divide/1
